simulink model "part2b_starter"  (R2024b)
settings: Solver=ode1  StartTime=0.0  StopTime=400  FixedStep=.002  RelTol=1e-3  EnableMultiTasking=on
InitFcn:
  | StartStop___PWM = 1
libraries: c2837xDlib x2, ece486lib x1
settings Model: SimulationMode=external  ExtModeTrigDuration=8  Creator=The MathWorks, Inc.  LastModifiedBy=fve2
settings SolverCC: AlgebraicLoopSolver=TrustRegion  MaxZcPerStep=1
settings OptimizationCC: DefaultUnderspecifiedDataType=single  EnhancedBackFolding=on  PassReuseOutputArgsAs=Individual arguments  MaxStackSize=1024  OptimizeBlockOrder=speed  DifferentSizesBufferReuse=on  OptimizationCustomize=off  EfficientTunableParamExpr=on
settings DebuggingCC: ParameterTunabilityLossMsg=error  UnconnectedInputMsg=warning  UnconnectedOutputMsg=warning  UnconnectedLineMsg=warning
settings HardwareCC: ProdBitPerChar=16  ProdBitPerInt=16  ProdBitPerPointer=32  ProdBitPerSizeT=32  ProdBitPerPtrDiffT=32  ProdLargestAtomicInteger=Integer  ProdLargestAtomicFloat=None  ProdWordSize=16  ProdLongLongMode=on  ProdHWDeviceType=Texas Instruments->C2000
settings ModelReferenceCC: EnableRefExpFcnMdlSchedulingChecks=on
settings SFSimCC: MATLABDynamicMemAlloc=off
settings RTWCC: Description=Embedded Coder  SystemTargetFile=ert.tlc  HardwareBoard=TI Delfino F28379D LaunchPad  TemplateMakefile=ert_default_tmf  GenerateReport=on  Toolchain=Texas Instruments Code Composer Studio (C2000)  GPUComputeCapability=3.5  DLArmComputeVersion=19.05
settings CodeAppCC: ForceParamTrailComments=on  IgnoreCustomStorageClasses=off  OperatorAnnotations=on  SimulinkDataObjDesc=on  SFDataObjDesc=on  InsertBlockDesc=on
settings ERTTargetCC: CodeReplacementLibrary=TI C28x  SupportContinuousTime=on  ExtModeStaticAllocSize=10000  InlinedParameterPlacement=Hierarchical  DynamicArrayContainerType=coder::array

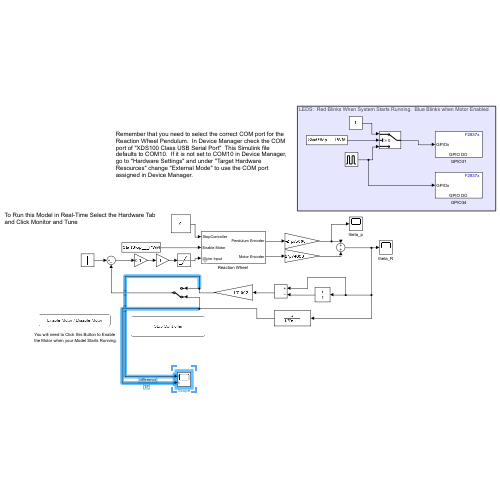
[thumbnail: Simulink's stored preview of the top-level diagram]
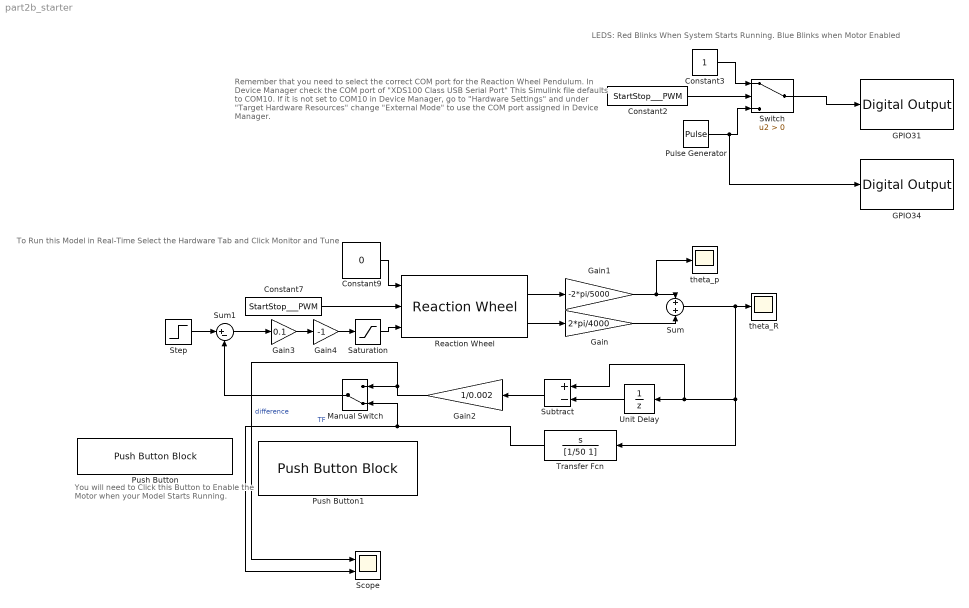
== system part2b_starter ==
  note: LEDS: Red Blinks When System Starts Running. Blue Blinks when Motor Enabled
  note: To Run this Model in Real-Time Select the Hardware Tab
      | and Click Monitor and Tune
  note: Remember that you need to select the correct COM port for the Reaction Wheel Pendulum. In Device Manager check the COM port of "XDS100 Class USB Serial Port" This Simulink file defaults to COM10. If it is not set to COM10 in Device Manager, go to "Hardware Settings" and under "Target Hardware Resources" change "External Mode" to use the COM port assigned in Device Manager.
  note: You will need to Click this Button to Enable
      | the Motor when your Model Starts Running.
  Constant2 : Constant  Value=StartStop___PWM
  Constant3 : Constant
  Constant7 : Constant  Value=StartStop___PWM
  Constant9 : Constant  Value=0
  GPIO31 : c2837xDlib/Digital Output  GPIO_Number=GPIO24~GPIO31  GPIO_Bit0=off  GPIO_BIT0_Toggle=off  GPIO_Bit1=off  GPIO_BIT1_Toggle=off  GPIO_Bit2=off  GPIO_BIT2_Toggle=off  GPIO_Bit3=off  GPIO_BIT3_Toggle=off  GPIO_Bit4=off  GPIO_BIT4_Toggle=off  GPIO_Bit5=off  GPIO_BIT5_Toggle=off  GPIO_Bit6=off  GPIO_BIT6_Toggle=off  GPIO_Bit7=on  GPIO_BIT7_Toggle=off
  GPIO34 : c2837xDlib/Digital Output  GPIO_Number=GPIO32~GPIO39  GPIO_Bit0=off  GPIO_BIT0_Toggle=off  GPIO_Bit1=off  GPIO_BIT1_Toggle=off  GPIO_Bit2=on  GPIO_BIT2_Toggle=off  GPIO_Bit3=off  GPIO_BIT3_Toggle=off  GPIO_Bit4=off  GPIO_BIT4_Toggle=off  GPIO_Bit5=off  GPIO_BIT5_Toggle=off  GPIO_Bit6=off  GPIO_BIT6_Toggle=off  GPIO_Bit7=off  GPIO_BIT7_Toggle=off
  Gain : Gain  Gain=2*pi/4000
  Gain1 : Gain  Gain=-2*pi/5000
  Gain2 : Gain  Gain=1/0.002
  Gain3 : Gain  Gain=0.1
  Gain4 : Gain  Gain=-1
  Manual Switch : ManualSwitch  CurrentSetting=0
  Pulse Generator : DiscretePulseGenerator  PulseType=Time based  Period=1  PulseWidth=50
  Push Button : PushButtonBlock  ButtonText=Enable Motor / Disable Motor  OnValue=0  ButtonType=Latch  OffValue=1.000000
  Push Button1 : PushButtonBlock  ButtonText=Stop Controller  OffValue=0.000000
  "Reaction Wheel " : ece486lib/Reaction Wheel  SampleTime=.002
  Saturation : Saturate  UpperLimit=10  LowerLimit=-10
  Scope : Scope  NumInputPorts=2
  Step : Step  After=100  SampleTime=0
  Subtract : Sum  Inputs=+-
  Sum : Sum
  Sum1 : Sum  Inputs=|+-
  Switch : Switch  Criteria=u2 > Threshold  SaturateOnIntegerOverflow=off  InputSameDT=off
  Transfer Fcn : TransferFcn  Numerator=[1 0]  Denominator=[1/50 1]
  Unit Delay : UnitDelay  SampleTime=0.002  HasFrameUpgradeWarning=on
  theta_R : Scope
  theta_p : Scope
  wires:
  Constant9/1 -> "Reaction Wheel "/1
  Constant7/1 -> "Reaction Wheel "/2
  Pulse Generator/1 -> GPIO34/1, Switch/3
  Switch/1 -> GPIO31/1
  Constant2/1 -> Switch/2
  Constant3/1 -> Switch/1
  "Reaction Wheel "/1 -> Gain1/1
  "Reaction Wheel "/2 -> Gain/1
  Gain1/1 -> theta_p/1, Sum/1
  Gain/1 -> Sum/2
  Subtract/1 -> Gain2/1
  Unit Delay/1 -> Subtract/2
  Sum/1 -> Transfer Fcn/1, Subtract/1, Unit Delay/1, theta_R/1
  Step/1 -> Sum1/1
  Saturation/1 -> "Reaction Wheel "/3
  Sum1/1 -> Gain3/1
  Gain2/1 -> Scope/1, Manual Switch/1  "difference"
  Transfer Fcn/1 -> Scope/2, Manual Switch/2  "TF"
  Manual Switch/1 -> Sum1/2
  Gain4/1 -> Saturation/1
  Gain3/1 -> Gain4/1
